simulink model "mCSControls_DG"  (R2012b)
settings: Solver=FixedStepDiscrete  StartTime=0.0  StopTime=10.0  RelTol=1e-3
values from neighbouring files (symbols this model uses):
  CDF2FThreshold = 45    [ControlCal_DG.m]
  CDF2TempThreshold = 20    [ControlCal_DG.m]
  delay = 5    [ControlCal_DG.m]
  DFThresh = 33    [ControlCal_DG.m]
  H = [90 90 90 90]    [ControlCal_DG.m]
  HeatTempThresh1 = 40    [ControlCal_DG.m]
  HeatTempThresh2 = 30    [ControlCal_DG.m]
  HeatTempThresh3 = 20    [ControlCal_DG.m]
  HStabilizationTime = 2*60    (= 120)    [ControlCal_DG.m]
  I_FAN = -1    [ControlCal_DG.m]
  I_VALVE = -1    [ControlCal_DG.m]
  initialSet = [1 1 1]    [ControlCal_DG.m]
  PBFTempThreshold = 30    [ControlCal_DG.m]
  PowerModeSwitchDelay = 30    [ControlCal_DG.m]
  SVocThresh = 550    [ControlCal_DG.m]
  T = [0 4 7 10]    [ControlCal_DG.m]
  Ts = 0.5    [ControlCal_DG.m]
  TSTempSetPoint = -2    [ControlCal_DG.m]
  TV1FThresh = 45    [ControlCal_DG.m]
  TV2FThresh = 60    [ControlCal_DG.m]
  VbatThresh = 22    [ControlCal_DG.m]
  VocDecRate = 0.5    [ControlCal_DG.m]
  VocIncrement = 5    [ControlCal_DG.m]
libraries: c2833xlib x29, simulink x23, c280xlib x11, idelinklib_tgtpref x1
(part 4 of 4)

== stateflow chart mCSControls_DG/Controls/Chart ==
  note: Variable 'count' is to find the time after the compressor has been switched off.
      | The heater is switched on if the time the compressor has been off > 45min.
      | Initally it's assigned a value > 45min to make sure heater runs at startup depending on ambient temp.
  state Running
    note: RelayOn is a global variable which controls when a relay can switch on.
        | This ensures only one relay switches on at a time and there is a 'delay' between multiple relays switching on.
    state StartupRelaysOff
      en,du:
      RelaysOP=RelaysOff;
      RelayOn=1;
      Pstatus=0;
    state PowerBatteryCheck
      en,du:
      [RelaysOP, Pstatus]=PowerModeSelection(RelaysOP,Inputs);
      count++;
    state PowerAvailable
      state PowerMonitor [parallel]
        settings: executionOrder=1
        state SolarPowerTesting
        state NormalOn
        note: Resetting TestVoc to threshold since it seems to run;
            | There is no guarantee TestVoc is the minimum Voc needed, it might be able to run at lower Voc too.
        state SwitchOff
          en,du: Pstatus=0;
        (default) -> NormalOn
        NormalOn -> SolarPowerTesting [order 2] : [RelaysOP.RS && Inputs.DriveParams.OP.OPFreq<DFThresh && RelaysOP.CRUN && CRUNOn]
        NormalOn -> NormalOn [order 1] : after(60,sec)[VocOffset>0]
            | {VocOffset=RelaysOP.RG*(VocOffset-VocDecRate)}
        SolarPowerTesting -> NormalOn [order 2] : after(20,sec){TestVoc = SVocThresh;}
        SolarPowerTesting -> SwitchOff [order 1] : after(20,sec)[powerSwitchCondition(RelaysOP, Inputs)]
        NormalOn -> SwitchOff [order 3] : [powerSwitchCondition(RelaysOP, Inputs)]
      state CompressorControl [parallel]
        settings: executionOrder=2
        state BeginCompressorOnSequence
        state switchOnHeater
          en:
          duration = heaterDuration(Inputs.Sensors.TA);
          du:
          RelaysOP.HEATER = 1;
        state SystemHeated
          en,du:
          RelaysOP.HEATER = 0;
          count = 0;
          CompOnCount = 0;
        state ValveCondenserCompressorControl
          state FanValveControl [parallel]
            settings: executionOrder=1
            note: FVOn ensures the Fault and Delay conditions in this substate are checked only when this valve switches on.
                | It is the local counterpart of the global variable RelayOn
            state FanValveOff
              en,du:
              RelaysOP.FV=0;
            state FanValveOn
              en:
              ILoadCurrent=Inputs.DCParams.Iload;
              RelaysOP.FV=1;
            state FanValveFault
              en:
              RelaysOP.FV=2;
            (default) -> Running.PowerAvailable.CompressorControl.ValveCondenserCompressorControl.FanValveControl.FanValveOff
            Running.PowerAvailable.CompressorControl.ValveCondenserCompressorControl.FanValveControl.FanValveOn -> Running.PowerAvailable.CompressorControl.ValveCondenserCompressorControl.FanValveControl.FanValveOff [order 1] : [~TempCondition(RelaysOP, Inputs)]{CompOnCount--; RelayOn=1;}
            Running.PowerAvailable.CompressorControl.ValveCondenserCompressorControl.FanValveControl.FanValveOff -> Running.PowerAvailable.CompressorControl.ValveCondenserCompressorControl.FanValveControl.FanValveOn : [RelayOn && TempCondition(RelaysOP, Inputs)]
                | {CompOnCount++; RelayOn=0;FVOn=0;}
            Running.PowerAvailable.CompressorControl.ValveCondenserCompressorControl.FanValveControl.FanValveOn -> Running.PowerAvailable.CompressorControl.ValveCondenserCompressorControl.FanValveControl.FanValveFault [order 3] : after(delay-1,sec)[~FVOn && Inputs.DCParams.Iload<ILoadCurrent+I_VALVE]{CompOnCount--; RelayOn=1;}
            Running.PowerAvailable.CompressorControl.ValveCondenserCompressorControl.FanValveControl.FanValveFault -> (junction 356) : after(105,sec){RelaysOP.FV=0}
            (junction 356) -> Running.PowerAvailable.CompressorControl.ValveCondenserCompressorControl.FanValveControl.FanValveOn : after(120,sec)[RelayOn]
                | {CompOnCount++; RelayOn=0; FVOn=0;}
            Running.PowerAvailable.CompressorControl.ValveCondenserCompressorControl.FanValveControl.FanValveOn -> Running.PowerAvailable.CompressorControl.ValveCondenserCompressorControl.FanValveControl.FanValveOn [order 2] : after(delay,sec)[~FVOn]{RelayOn=1; FVOn=1;}
          state ThermalStorageValve1Control [parallel]
            settings: executionOrder=2
            note: TV1On ensures the Fault and Delay conditions in this substate are checked only when this valve switches on.
                | It is the local counterpart of the global variable RelayOn
            state TV1ValveOff
              en,du:
              RelaysOP.TV1=0;
            state TESValveOn
              en,du:
              RelaysOP.TV1=1;
            (default) -> TV1ValveOff
            TESValveOn -> TV1ValveOff [order 1] : [~TV1TempOnCondition(RelaysOP, Inputs)]
                | {CompOnCount--; RelayOn=1;}
            TV1ValveOff -> TESValveOn : [RelayOn && TV1TempOnCondition(RelaysOP, Inputs)]
                | {CompOnCount++; RelayOn=0; TV1On=0;}
            TESValveOn -> TESValveOn [order 2] : after(delay,sec)[~TV1On]{RelayOn=1; TV1On=1;}
          state CompAndCondenserFan1Control [parallel]
            settings: executionOrder=3
            note: CDF1On and CRUNOn ensures the Fault and Delay conditions in this substate are checked only when this valve switches on.
                | It is the local counterpart of the global variable RelayOn
            state CompCondenserOff
              en,du:
              RelaysOP.CRUN=0;
              RelaysOP.RG2=0;
              RelaysOP.CDF1=0;
              count++;
            state CondenserFan1Fault
              en:
              RelaysOP.CDF1=2;
            state CondenserFan1On
              en:
              ILoadCurrent=Inputs.DCParams.Iload;
              RelaysOP.CDF1=1;
            state CompOn
              en: TestVoc = Inputs.DCParams.Voc
              du:
              RelaysOP.CRUN=1;
              count=0;
            (default) -> Running.PowerAvailable.CompressorControl.ValveCondenserCompressorControl.CompAndCondenserFan1Control.CompCondenserOff
            Running.PowerAvailable.CompressorControl.ValveCondenserCompressorControl.CompAndCondenserFan1Control.CompOn -> Running.PowerAvailable.CompressorControl.ValveCondenserCompressorControl.CompAndCondenserFan1Control.CompCondenserOff [order 2] : [CompOnCount==0]{RelayOn=1;}
            Running.PowerAvailable.CompressorControl.ValveCondenserCompressorControl.CompAndCondenserFan1Control.CompCondenserOff -> Running.PowerAvailable.CompressorControl.ValveCondenserCompressorControl.CompAndCondenserFan1Control.CondenserFan1On : [RelayOn && CompOnCount>0]
                | {RelayOn=0; CDF1On=0;}
            Running.PowerAvailable.CompressorControl.ValveCondenserCompressorControl.CompAndCondenserFan1Control.CondenserFan1On -> Running.PowerAvailable.CompressorControl.ValveCondenserCompressorControl.CompAndCondenserFan1Control.CondenserFan1Fault [order 3] : after(delay-1,sec)[~CDF1On && Inputs.DCParams.Iload<ILoadCurrent+I_FAN]{ RelayOn=1;}
            Running.PowerAvailable.CompressorControl.ValveCondenserCompressorControl.CompAndCondenserFan1Control.CondenserFan1On -> Running.PowerAvailable.CompressorControl.ValveCondenserCompressorControl.CompAndCondenserFan1Control.CondenserFan1On [order 1] : after(delay, sec)[~CDF1On]{RelayOn=1; CDF1On=1;}
            Running.PowerAvailable.CompressorControl.ValveCondenserCompressorControl.CompAndCondenserFan1Control.CondenserFan1Fault -> (junction 647) : after(105,sec){RelaysOP.CDF1=0;}
            (junction 647) -> Running.PowerAvailable.CompressorControl.ValveCondenserCompressorControl.CompAndCondenserFan1Control.CondenserFan1On : after(120,sec)[RelayOn]
                | {RelayOn=0; CDF1On=0;}
            Running.PowerAvailable.CompressorControl.ValveCondenserCompressorControl.CompAndCondenserFan1Control.CondenserFan1On -> Running.PowerAvailable.CompressorControl.ValveCondenserCompressorControl.CompAndCondenserFan1Control.CompOn [order 2] : [RelayOn]{RelayOn=0; CRUNOn=0;}
            Running.PowerAvailable.CompressorControl.ValveCondenserCompressorControl.CompAndCondenserFan1Control.CompOn -> Running.PowerAvailable.CompressorControl.ValveCondenserCompressorControl.CompAndCondenserFan1Control.CompOn [order 1] : after(1, sec)[~CRUNOn]
                | {RelayOn=1; CRUNOn=1; RelaysOP.RG2=RelaysOP.RG;}
          state CondenserFan2Control [parallel]
            settings: executionOrder=4
            note: CDF2On ensures the Fault and Delay conditions in this substate are checked only when this valve switches on.
                | It is the local counterpart of the global variable RelayOn
            state CondenserFan2Off
              en,du:
              RelaysOP.CDF2=0;
            state CondenserFan2Fault
              en:
              RelaysOP.CDF2=2;
            state CondenserFan2On
              en,du:
              ILoadCurrent=Inputs.DCParams.Iload;
              RelaysOP.CDF2=1;
            (default) -> Running.PowerAvailable.CompressorControl.ValveCondenserCompressorControl.CondenserFan2Control.CondenserFan2Off
            Running.PowerAvailable.CompressorControl.ValveCondenserCompressorControl.CondenserFan2Control.CondenserFan2On -> Running.PowerAvailable.CompressorControl.ValveCondenserCompressorControl.CondenserFan2Control.CondenserFan2Off [order 1] : [~CDF2Condition(RelaysOP, Inputs)]{RelayOn=1;}
            Running.PowerAvailable.CompressorControl.ValveCondenserCompressorControl.CondenserFan2Control.CondenserFan2Off -> Running.PowerAvailable.CompressorControl.ValveCondenserCompressorControl.CondenserFan2Control.CondenserFan2On : [RelayOn && CDF2Condition(RelaysOP, Inputs)]
                | {RelayOn=0; CDF2On=0;}
            Running.PowerAvailable.CompressorControl.ValveCondenserCompressorControl.CondenserFan2Control.CondenserFan2On -> Running.PowerAvailable.CompressorControl.ValveCondenserCompressorControl.CondenserFan2Control.CondenserFan2Fault [order 3] : after(delay-1,sec)[~CDF2On && Inputs.DCParams.Iload<ILoadCurrent+I_FAN]{ RelayOn=1;}
            Running.PowerAvailable.CompressorControl.ValveCondenserCompressorControl.CondenserFan2Control.CondenserFan2Fault -> (junction 433) : after(105,sec){RelaysOP.CDF2=0;}
            (junction 433) -> Running.PowerAvailable.CompressorControl.ValveCondenserCompressorControl.CondenserFan2Control.CondenserFan2On : after(120,sec)[RelayOn]
                | {RelayOn=0; CDF2On=0;}
            Running.PowerAvailable.CompressorControl.ValveCondenserCompressorControl.CondenserFan2Control.CondenserFan2On -> Running.PowerAvailable.CompressorControl.ValveCondenserCompressorControl.CondenserFan2Control.CondenserFan2On [order 2] : after(delay,sec)[~CDF2On]{RelayOn=1; CDF2On=1;}
          note: CompOnCount keeps count of how many relays are On.
              | If it is greater than 1, the compressor switches on.
        (default) -> Running.PowerAvailable.CompressorControl.BeginCompressorOnSequence
        Running.PowerAvailable.CompressorControl.ValveCondenserCompressorControl -> Running.PowerAvailable.CompressorControl.BeginCompressorOnSequence : [count>2700/Ts]
        Running.PowerAvailable.CompressorControl.BeginCompressorOnSequence -> Running.PowerAvailable.CompressorControl.SystemHeated [order 2] : after(delay,sec)
        Running.PowerAvailable.CompressorControl.BeginCompressorOnSequence -> Running.PowerAvailable.CompressorControl.switchOnHeater [order 1] : [Inputs.Sensors.TA<HeatTempThresh1 && count>2700/Ts]
        Running.PowerAvailable.CompressorControl.switchOnHeater -> Running.PowerAvailable.CompressorControl.SystemHeated : after(duration, sec)
        Running.PowerAvailable.CompressorControl.SystemHeated -> Running.PowerAvailable.CompressorControl.ValveCondenserCompressorControl : after(delay, sec)
      state HumidityControl [parallel]
        settings: executionOrder=3
        state HumidityPumpOff
          en,du:
          RelaysOP.PUMP=0;
          RelaysOP.PV=0;
        note: HOn ensures the Fault and Delay conditions in this substate are checked only when this valve switches on.
            | It is the local counterpart of the global variable RelayOn
        state HumidityPumpOn
          en,du:
          RelaysOP.PV=1;
          RelaysOP.PUMP=1;
        (default) -> Running.PowerAvailable.HumidityControl.HumidityPumpOff
        Running.PowerAvailable.HumidityControl.HumidityPumpOn -> Running.PowerAvailable.HumidityControl.HumidityPumpOff [order 2] : [~HCondition(Inputs)]{RelayOn=1;}
        Running.PowerAvailable.HumidityControl.HumidityPumpOff -> Running.PowerAvailable.HumidityControl.HumidityPumpOn : [RelayOn && HCondition(Inputs)]
            | {RelayOn=0; HOn=0;}
        Running.PowerAvailable.HumidityControl.HumidityPumpOn -> Running.PowerAvailable.HumidityControl.HumidityPumpOn [order 1] : after(delay,sec)[~HOn]{RelayOn=1; HOn=1;}
      state FanControl [parallel]
        settings: executionOrder=4
        state FanOff
          en,du:
          RelaysOP.F1=0
          RelaysOP.F2=0;
        note: FOn ensures the Fault and Delay conditions in this substate are checked only when this valve switches on.
            | It is the local counterpart of the global variable RelayOn
        state FanFault
          en:
          RelaysOP.F1=2;
          RelaysOP.F2=2;
        state Fan2Off
          en,du:
          ILoadCurrent=Inputs.DCParams.Iload;
          RelaysOP.F1=1;
          RelaysOP.F2=0;
        state FansOn
          en,du:
          RelaysOP.F1=1;
          RelaysOP.F2=1;
        (default) -> Running.PowerAvailable.FanControl.FanOff
        Running.PowerAvailable.FanControl.Fan2Off -> Running.PowerAvailable.FanControl.FanOff [order 1] : [~RelaysOP.FV]{RelayOn=1;}
        Running.PowerAvailable.FanControl.FanOff -> Running.PowerAvailable.FanControl.Fan2Off : [RelayOn && RelaysOP.FV==1]
            | {RelayOn=0; FOn=0;}
        Running.PowerAvailable.FanControl.Fan2Off -> Running.PowerAvailable.FanControl.FanFault [order 3] : after(delay-1,sec)[~FOn && Inputs.DCParams.Iload<ILoadCurrent+I_FAN]{ RelayOn=1;}
        Running.PowerAvailable.FanControl.Fan2Off -> Running.PowerAvailable.FanControl.FansOn [order 4] : after(3*60,sec)[RelaysOP.FV==1]
        Running.PowerAvailable.FanControl.FanFault -> (junction 439) : after(105,sec){RelaysOP.F1=0; RelaysOP.F2=0;}
        (junction 439) -> Running.PowerAvailable.FanControl.Fan2Off : after(120,sec)[RelayOn]
            | {RelayOn=0; FOn=0;}
        Running.PowerAvailable.FanControl.FansOn -> Running.PowerAvailable.FanControl.Fan2Off : after(1*60,sec)
        Running.PowerAvailable.FanControl.Fan2Off -> Running.PowerAvailable.FanControl.Fan2Off [order 2] : after(delay,sec)[~FOn]{RelayOn=1; FOn=1;}
      state PanelBoxFanControl [parallel]
        settings: executionOrder=5
        state PanelBoxFanOff
          en,du:
          RelaysOP.PBF=0
        note: PBFOn ensures the Fault and Delay conditions in this substate are checked only when this valve switches on.
            | It is the local counterpart of the global variable RelayOn
        note: 0.5 is for Hysteresis in temperature control
        state PanelBoxFanOn
          en,du:
          RelaysOP.PBF=1;
        (default) -> Running.PowerAvailable.PanelBoxFanControl.PanelBoxFanOff
        Running.PowerAvailable.PanelBoxFanControl.PanelBoxFanOn -> Running.PowerAvailable.PanelBoxFanControl.PanelBoxFanOff [order 1] : [Inputs.Sensors.TA<PBFTempThreshold-0.5]{RelayOn=1;}
        Running.PowerAvailable.PanelBoxFanControl.PanelBoxFanOff -> Running.PowerAvailable.PanelBoxFanControl.PanelBoxFanOn : [RelayOn && Inputs.Sensors.TA>PBFTempThreshold]
            | {RelayOn=0; PBFOn=0;}
        Running.PowerAvailable.PanelBoxFanControl.PanelBoxFanOn -> Running.PowerAvailable.PanelBoxFanControl.PanelBoxFanOn [order 2] : after(delay,sec)[~PBFOn]{RelayOn=1; PBFOn=1;}
    state RelaysOff
      en,du:
      RelaysOP=RelaysOff;
      RelayOn=1;
    state BatteryAvailable
      state PowerMonitor [parallel]
        settings: executionOrder=1
        state PowerNotAvailable
          en,du: count++
        state PowerAvailable
          en,du: Pstatus=1;
        (default) -> Running.BatteryAvailable.PowerMonitor.PowerNotAvailable
        Running.BatteryAvailable.PowerMonitor.PowerNotAvailable -> Running.BatteryAvailable.PowerMonitor.PowerNotAvailable [order 2] : after(60,sec)[VocOffset>0]
            | {VocOffset=VocOffset-VocDecRate}
        Running.BatteryAvailable.PowerMonitor.PowerNotAvailable -> Running.BatteryAvailable.PowerMonitor.PowerAvailable [order 1] : [powerOnCondition(RelaysOP, Inputs)]
      state HumidityControl [parallel]
        settings: executionOrder=2
        state HumidityPumpOff
          en,du:
          RelaysOP.PUMP=0;
          RelaysOP.PV=0;
        note: HOn ensures the Fault and Delay conditions in this substate are checked only when this valve switches on.
            | It is the local counterpart of the global variable RelayOn
        state HumidityPumpOn
          en,du:
          RelaysOP.PV=1;
          RelaysOP.PUMP=1;
        (default) -> Running.BatteryAvailable.HumidityControl.HumidityPumpOff
        Running.BatteryAvailable.HumidityControl.HumidityPumpOn -> Running.BatteryAvailable.HumidityControl.HumidityPumpOff [order 2] : [~HCondition(Inputs)]{RelayOn=1;}
        Running.BatteryAvailable.HumidityControl.HumidityPumpOff -> Running.BatteryAvailable.HumidityControl.HumidityPumpOn : [RelayOn && HCondition(Inputs)]
            | {RelayOn=0; HOn=0;}
        Running.BatteryAvailable.HumidityControl.HumidityPumpOn -> Running.BatteryAvailable.HumidityControl.HumidityPumpOn [order 1] : after(delay,sec)[~HOn]{RelayOn=1; HOn=1;}
      state FanControl [parallel]
        settings: executionOrder=3
        (history)
        note: FOn ensures the Fault and Delay conditions in this substate are checked only when this valve switches on.
            | It is the local counterpart of the global variable RelayOn
        state FanOff
          en,du:
          RelaysOP.F1=0
          RelaysOP.F2=0;
        state FanConditionalOff
          en,du:
          RelaysOP.F1=0;
          RelaysOP.F2=0;
        state FanConditionalOn
          en:CurrentH1Temp=Inputs.Sensors.TH1;
          du:
          RelaysOP.F1=1;
          RelaysOP.F2=0;
        note: In Battery Mode, if Temperature of the Holding is greater than setpoint,
            | switch on the fan, wait for 5 min to see if temp reduces, but if not,
            | switch off the fan.
        (default) -> Running.BatteryAvailable.FanControl.FanOff
        Running.BatteryAvailable.FanControl.FanOff -> FanConditionalOn : [RelayOn && TempCheck(RelaysOP, Inputs)]
            | {RelayOn=0; FOn=0;}
        FanConditionalOff -> Running.BatteryAvailable.FanControl.FanOff [order 1] : [~TempCheck(RelaysOP, Inputs)]{RelayOn=1;}
        FanConditionalOn -> Running.BatteryAvailable.FanControl.FanOff [order 1] : [~TempCheck(RelaysOP, Inputs)]{RelayOn=1;}
        FanConditionalOn -> FanConditionalOff [order 3] : after(5*60,sec)
            | [Inputs.Sensors.TH1>CurrentH1Temp]
        FanConditionalOff -> FanConditionalOn [order 2] : after(4*60,sec)
        FanConditionalOn -> FanConditionalOn [order 2] : after(delay,sec)[~FOn]{RelayOn=1; FOn=1;}
      state PanelBoxFanControl [parallel]
        settings: executionOrder=4
        state PanelBoxFanOff
          en,du:
          RelaysOP.PBF=0
        note: PBFOn ensures the Fault and Delay conditions in this substate are checked only when this valve switches on.
            | It is the local counterpart of the global variable RelayOn
        note: 0.5 is for Hysteresis in temperature control
        state PanelBoxFanOn
          en,du:
          RelaysOP.PBF=1;
        (default) -> Running.BatteryAvailable.PanelBoxFanControl.PanelBoxFanOff
        Running.BatteryAvailable.PanelBoxFanControl.PanelBoxFanOn -> Running.BatteryAvailable.PanelBoxFanControl.PanelBoxFanOff [order 1] : [Inputs.Sensors.TA<PBFTempThreshold-0.5]{RelayOn=1;}
        Running.BatteryAvailable.PanelBoxFanControl.PanelBoxFanOff -> Running.BatteryAvailable.PanelBoxFanControl.PanelBoxFanOn : [RelayOn && Inputs.Sensors.TA>PBFTempThreshold]
            | {RelayOn=0; PBFOn=0;}
        Running.BatteryAvailable.PanelBoxFanControl.PanelBoxFanOn -> Running.BatteryAvailable.PanelBoxFanControl.PanelBoxFanOn [order 2] : after(delay,sec)[~PBFOn]{RelayOn=1; PBFOn=1;}
    state DieselMode
      state PowerMonitor [parallel]
        settings: executionOrder=1
        state TestingDG
        state PowerNotAvailable
        state SwitchOffDiesel
          en,du: RelaysOP.DGOFF=1;
        state PowerAvailable
          en,du:
          RelaysOP.DGOFF=0;
          Pstatus=1;
        (default) -> Running.DieselMode.PowerMonitor.PowerNotAvailable
        Running.DieselMode.PowerMonitor.PowerNotAvailable -> TestingDG [order 3] : [RelaysOP.CRUN==1 && Inputs.DriveParams.OP.OPFreq<DFThresh]
        Running.DieselMode.PowerMonitor.PowerNotAvailable -> Running.DieselMode.PowerMonitor.PowerNotAvailable [order 2] : after(60,sec)[VocOffset>0]
            | {VocOffset=VocOffset-VocDecRate}
        TestingDG -> Running.DieselMode.PowerMonitor.PowerNotAvailable [order 1] : after(20,sec)[Inputs.DriveParams.OP.OPFreq>DFThresh]
        TestingDG -> SwitchOffDiesel [order 2] : after(20,sec)
        Running.DieselMode.PowerMonitor.PowerNotAvailable -> SwitchOffDiesel [order 1] : [powerOnCondition(RelaysOP, Inputs) || Inputs.DCParams.Vbat<VbatThresh]
        SwitchOffDiesel -> Running.DieselMode.PowerMonitor.PowerAvailable : after(4,sec)
      state CompressorControl [parallel]
        settings: executionOrder=2
        state BeginCompressorOnSequence
        state switchOnHeater
          en:
          duration = heaterDuration(Inputs.Sensors.TA);
          du:
          RelaysOP.HEATER = 1;
        state SystemHeated
          en,du:
          RelaysOP.HEATER = 0;
          count = 0;
          CompOnCount = 0;
        state ValveCondenserCompressorControl
          state FanValveControl [parallel]
            settings: executionOrder=1
            note: FVOn ensures the Fault and Delay conditions in this substate are checked only when this valve switches on.
                | It is the local counterpart of the global variable RelayOn
            state FanValveOff
              en,du:
              RelaysOP.FV=0;
            state FanValveOn
              en:
              ILoadCurrent=Inputs.DCParams.Iload;
              RelaysOP.FV=1;
            state FanValveFault
              en:
              RelaysOP.FV=2;
            (default) -> Running.DieselMode.CompressorControl.ValveCondenserCompressorControl.FanValveControl.FanValveOff
            Running.DieselMode.CompressorControl.ValveCondenserCompressorControl.FanValveControl.FanValveOn -> Running.DieselMode.CompressorControl.ValveCondenserCompressorControl.FanValveControl.FanValveOff [order 1] : [~TempCondition(RelaysOP, Inputs)]{CompOnCount--; RelayOn=1;}
            Running.DieselMode.CompressorControl.ValveCondenserCompressorControl.FanValveControl.FanValveOff -> Running.DieselMode.CompressorControl.ValveCondenserCompressorControl.FanValveControl.FanValveOn : [RelayOn && TempCondition(RelaysOP, Inputs)]
                | {CompOnCount++; RelayOn=0;FVOn=0;}
            Running.DieselMode.CompressorControl.ValveCondenserCompressorControl.FanValveControl.FanValveOn -> Running.DieselMode.CompressorControl.ValveCondenserCompressorControl.FanValveControl.FanValveFault [order 3] : after(delay-1,sec)[~FVOn && Inputs.DCParams.Iload<ILoadCurrent+I_VALVE]{CompOnCount--; RelayOn=1;}
            Running.DieselMode.CompressorControl.ValveCondenserCompressorControl.FanValveControl.FanValveFault -> (junction 796) : after(105,sec){RelaysOP.FV=0}
            (junction 796) -> Running.DieselMode.CompressorControl.ValveCondenserCompressorControl.FanValveControl.FanValveOn : after(120,sec)[RelayOn]
                | {CompOnCount++; RelayOn=0; FVOn=0;}
            Running.DieselMode.CompressorControl.ValveCondenserCompressorControl.FanValveControl.FanValveOn -> Running.DieselMode.CompressorControl.ValveCondenserCompressorControl.FanValveControl.FanValveOn [order 2] : after(delay,sec)[~FVOn]{RelayOn=1; FVOn=1;}
          state CompAndCondenserFan1Control [parallel]
            settings: executionOrder=2
            state CompCondenserOff
              en,du:
              RelaysOP.DGOFF=0;
              RelaysOP.RDG1=0;
              RelaysOP.CRUN=0;
              RelaysOP.RG2=0;
              RelaysOP.CDF1=0;
              count++;
            note: CDF1On and CRUNOn ensures the Fault and Delay conditions in this substate are checked only when this valve switches on.
                | It is the local counterpart of the global variable RelayOn
            state CondenserFan1Fault
              en:
              RelaysOP.CDF1=2;
            state CondenserFan1On
              en:
              ILoadCurrent=Inputs.DCParams.Iload;
              RelaysOP.CDF1=1;
            state DieselOff
              en,du:
              RelaysOP.DGOFF=1;
            state DieselOn
              en,du:
              RelaysOP.DGON=1;
              RelaysOP.RDG1=1;
            state CompOn
              en,du:
              RelaysOP.DGON=0;
              RelaysOP.CRUN=1;
              count=0;
            (default) -> Running.DieselMode.CompressorControl.ValveCondenserCompressorControl.CompAndCondenserFan1Control.CompCondenserOff
            Running.DieselMode.CompressorControl.ValveCondenserCompressorControl.CompAndCondenserFan1Control.DieselOff -> Running.DieselMode.CompressorControl.ValveCondenserCompressorControl.CompAndCondenserFan1Control.CompCondenserOff : after(4,sec)
            Running.DieselMode.CompressorControl.ValveCondenserCompressorControl.CompAndCondenserFan1Control.CompCondenserOff -> Running.DieselMode.CompressorControl.ValveCondenserCompressorControl.CompAndCondenserFan1Control.CondenserFan1On : [RelayOn && CompOnCount>0]
                | {RelayOn=0; CDF1On=0;}
            Running.DieselMode.CompressorControl.ValveCondenserCompressorControl.CompAndCondenserFan1Control.CondenserFan1On -> Running.DieselMode.CompressorControl.ValveCondenserCompressorControl.CompAndCondenserFan1Control.CondenserFan1Fault [order 3] : after(delay-1,sec)[~CDF1On && Inputs.DCParams.Iload<ILoadCurrent+I_FAN]{ RelayOn=1;}
            Running.DieselMode.CompressorControl.ValveCondenserCompressorControl.CompAndCondenserFan1Control.CondenserFan1On -> Running.DieselMode.CompressorControl.ValveCondenserCompressorControl.CompAndCondenserFan1Control.CondenserFan1On [order 1] : after(delay, sec)[~CDF1On]{RelayOn=1; CDF1On=1;}
            Running.DieselMode.CompressorControl.ValveCondenserCompressorControl.CompAndCondenserFan1Control.CondenserFan1Fault -> (junction 825) : after(105,sec){RelaysOP.CDF1=0;}
            (junction 825) -> Running.DieselMode.CompressorControl.ValveCondenserCompressorControl.CompAndCondenserFan1Control.CondenserFan1On : after(120,sec)[RelayOn]
                | {RelayOn=0; CDF1On=0;}
            Running.DieselMode.CompressorControl.ValveCondenserCompressorControl.CompAndCondenserFan1Control.CondenserFan1On -> Running.DieselMode.CompressorControl.ValveCondenserCompressorControl.CompAndCondenserFan1Control.DieselOn [order 2] : [RelayOn]{RelayOn=0; CRUNOn=0;}
            Running.DieselMode.CompressorControl.ValveCondenserCompressorControl.CompAndCondenserFan1Control.CompOn -> Running.DieselMode.CompressorControl.ValveCondenserCompressorControl.CompAndCondenserFan1Control.DieselOff [order 2] : [CompOnCount==0]{RelayOn=1;}
            Running.DieselMode.CompressorControl.ValveCondenserCompressorControl.CompAndCondenserFan1Control.DieselOn -> Running.DieselMode.CompressorControl.ValveCondenserCompressorControl.CompAndCondenserFan1Control.CompOn : after(4,sec)
            Running.DieselMode.CompressorControl.ValveCondenserCompressorControl.CompAndCondenserFan1Control.CompOn -> Running.DieselMode.CompressorControl.ValveCondenserCompressorControl.CompAndCondenserFan1Control.CompOn [order 1] : after(1, sec)[~CRUNOn]
                | {RelayOn=1; CRUNOn=1; RelaysOP.RG2=1;}
          state CondenserFan2Control [parallel]
            settings: executionOrder=3
            note: CDF2On ensures the Fault and Delay conditions in this substate are checked only when this valve switches on.
                | It is the local counterpart of the global variable RelayOn
            state CondenserFan2Off
              en,du:
              RelaysOP.CDF2=0;
            state CondenserFan2Fault
              en:
              RelaysOP.CDF2=2;
            state CondenserFan2On
              en,du:
              ILoadCurrent=Inputs.DCParams.Iload;
              RelaysOP.CDF2=1;
            (default) -> Running.DieselMode.CompressorControl.ValveCondenserCompressorControl.CondenserFan2Control.CondenserFan2Off
            Running.DieselMode.CompressorControl.ValveCondenserCompressorControl.CondenserFan2Control.CondenserFan2On -> Running.DieselMode.CompressorControl.ValveCondenserCompressorControl.CondenserFan2Control.CondenserFan2Off [order 1] : [~CDF2Condition(RelaysOP, Inputs)]{RelayOn=1;}
            Running.DieselMode.CompressorControl.ValveCondenserCompressorControl.CondenserFan2Control.CondenserFan2Off -> Running.DieselMode.CompressorControl.ValveCondenserCompressorControl.CondenserFan2Control.CondenserFan2On : [RelayOn && CDF2Condition(RelaysOP, Inputs)]
                | {RelayOn=0; CDF2On=0;}
            Running.DieselMode.CompressorControl.ValveCondenserCompressorControl.CondenserFan2Control.CondenserFan2On -> Running.DieselMode.CompressorControl.ValveCondenserCompressorControl.CondenserFan2Control.CondenserFan2Fault [order 3] : after(delay-1,sec)[~CDF2On && Inputs.DCParams.Iload<ILoadCurrent+I_FAN]{ RelayOn=1;}
            Running.DieselMode.CompressorControl.ValveCondenserCompressorControl.CondenserFan2Control.CondenserFan2Fault -> (junction 841) : after(105,sec){RelaysOP.CDF2=0;}
            (junction 841) -> Running.DieselMode.CompressorControl.ValveCondenserCompressorControl.CondenserFan2Control.CondenserFan2On : after(120,sec)[RelayOn]
                | {RelayOn=0; CDF2On=0;}
            Running.DieselMode.CompressorControl.ValveCondenserCompressorControl.CondenserFan2Control.CondenserFan2On -> Running.DieselMode.CompressorControl.ValveCondenserCompressorControl.CondenserFan2Control.CondenserFan2On [order 2] : after(delay,sec)[~CDF2On]{RelayOn=1; CDF2On=1;}
          note: CompOnCount keeps count of how many relays are On.
              | If it is greater than 1, the compressor switches on.
        (default) -> Running.DieselMode.CompressorControl.BeginCompressorOnSequence
        Running.DieselMode.CompressorControl.ValveCondenserCompressorControl -> Running.DieselMode.CompressorControl.BeginCompressorOnSequence : [count>2700/Ts]
        Running.DieselMode.CompressorControl.BeginCompressorOnSequence -> Running.DieselMode.CompressorControl.SystemHeated [order 2] : after(delay,sec)
        Running.DieselMode.CompressorControl.BeginCompressorOnSequence -> Running.DieselMode.CompressorControl.switchOnHeater [order 1] : [Inputs.Sensors.TA<HeatTempThresh1 && count>2700/Ts]
        Running.DieselMode.CompressorControl.switchOnHeater -> Running.DieselMode.CompressorControl.SystemHeated : after(duration, sec)
        Running.DieselMode.CompressorControl.SystemHeated -> Running.DieselMode.CompressorControl.ValveCondenserCompressorControl : after(delay, sec)
      state HumidityControl [parallel]
        settings: executionOrder=3
        state HumidityPumpOff
          en,du:
          RelaysOP.PUMP=0;
          RelaysOP.PV=0;
        note: HOn ensures the Fault and Delay conditions in this substate are checked only when this valve switches on.
            | It is the local counterpart of the global variable RelayOn
        state HumidityPumpOn
          en,du:
          RelaysOP.PV=1;
          RelaysOP.PUMP=1;
        (default) -> Running.DieselMode.HumidityControl.HumidityPumpOff
        Running.DieselMode.HumidityControl.HumidityPumpOn -> Running.DieselMode.HumidityControl.HumidityPumpOff [order 2] : [~HCondition(Inputs)]{RelayOn=1;}
        Running.DieselMode.HumidityControl.HumidityPumpOff -> Running.DieselMode.HumidityControl.HumidityPumpOn : [RelayOn && HCondition(Inputs)]
            | {RelayOn=0; HOn=0;}
        Running.DieselMode.HumidityControl.HumidityPumpOn -> Running.DieselMode.HumidityControl.HumidityPumpOn [order 1] : after(delay,sec)[~HOn]{RelayOn=1; HOn=1;}
      state FanControl [parallel]
        settings: executionOrder=4
        state FanOff
          en,du:
          RelaysOP.F1=0
          RelaysOP.F2=0;
        note: FOn ensures the Fault and Delay conditions in this substate are checked only when this valve switches on.
            | It is the local counterpart of the global variable RelayOn
        state FanFault
          en:
          RelaysOP.F1=2;
          RelaysOP.F2=2;
        state Fan2Off
          en,du:
          ILoadCurrent=Inputs.DCParams.Iload;
          RelaysOP.F1=1;
          RelaysOP.F2=0;
        state FansOn
          en,du:
          RelaysOP.F1=1;
          RelaysOP.F2=1;
        (default) -> Running.DieselMode.FanControl.FanOff
        Running.DieselMode.FanControl.Fan2Off -> Running.DieselMode.FanControl.FanOff [order 1] : [~RelaysOP.FV]{RelayOn=1;}
        Running.DieselMode.FanControl.FanOff -> Running.DieselMode.FanControl.Fan2Off : [RelayOn && RelaysOP.FV==1]
            | {RelayOn=0; FOn=0;}
        Running.DieselMode.FanControl.Fan2Off -> Running.DieselMode.FanControl.FanFault [order 3] : after(delay-1,sec)[~FOn && Inputs.DCParams.Iload<ILoadCurrent+I_FAN]{ RelayOn=1;}
        Running.DieselMode.FanControl.Fan2Off -> Running.DieselMode.FanControl.FansOn [order 4] : after(3*60,sec)[RelaysOP.FV==1]
        Running.DieselMode.FanControl.FanFault -> (junction 926) : after(105,sec){RelaysOP.F1=0; RelaysOP.F2=0;}
        (junction 926) -> Running.DieselMode.FanControl.Fan2Off : after(120,sec)[RelayOn]
            | {RelayOn=0; FOn=0;}
        Running.DieselMode.FanControl.FansOn -> Running.DieselMode.FanControl.Fan2Off : after(1*60,sec)
        Running.DieselMode.FanControl.Fan2Off -> Running.DieselMode.FanControl.Fan2Off [order 2] : after(delay,sec)[~FOn]{RelayOn=1; FOn=1;}
      state PanelBoxFanControl [parallel]
        settings: executionOrder=5
        state PanelBoxFanOff
          en,du:
          RelaysOP.PBF=0
        note: PBFOn ensures the Fault and Delay conditions in this substate are checked only when this valve switches on.
            | It is the local counterpart of the global variable RelayOn
        note: PBF always on in DG mode to cool rectifier
        state PanelBoxFanOn
          en,du:
          RelaysOP.PBF=1;
        (default) -> Running.DieselMode.PanelBoxFanControl.PanelBoxFanOff
        Running.DieselMode.PanelBoxFanControl.PanelBoxFanOff -> Running.DieselMode.PanelBoxFanControl.PanelBoxFanOn : [RelayOn]
            | {RelayOn=0; PBFOn=0;}
        Running.DieselMode.PanelBoxFanControl.PanelBoxFanOn -> Running.DieselMode.PanelBoxFanControl.PanelBoxFanOn : after(delay,sec)[~PBFOn]{RelayOn=1; PBFOn=1;}
      state BatteryChargeControl [parallel]
        settings: executionOrder=6
        state BatteryChargerOff
          en,du:
          RelaysOP.DGBATCHG=0
        state DieselOn
          en,du:
          RelaysOP.DGBATCHG=0;
        state BatteryChargerOn
          en,du:
          RelaysOP.DGBATCHG=1;
        (default) -> Running.DieselMode.BatteryChargeControl.BatteryChargerOff
        Running.DieselMode.BatteryChargeControl.BatteryChargerOn -> Running.DieselMode.BatteryChargeControl.BatteryChargerOff : [Inputs.DriveParams.OP.OPFreq<DFThresh]
        Running.DieselMode.BatteryChargeControl.DieselOn -> Running.DieselMode.BatteryChargeControl.BatteryChargerOff [order 2] : [Inputs.DriveParams.OP.OPFreq<DFThresh]
        Running.DieselMode.BatteryChargeControl.BatteryChargerOff -> Running.DieselMode.BatteryChargeControl.DieselOn : [Inputs.DriveParams.OP.OPFreq>DFThresh]
        Running.DieselMode.BatteryChargeControl.DieselOn -> Running.DieselMode.BatteryChargeControl.BatteryChargerOn [order 1] : after(30,sec)
    state DGBatteryChargeControl
      state DieselOn
        en,du:
        RelaysOP.DGON=1
        RelaysOP.DGBATCHG=0
      state BatteryChargerOn
        en,du:
        RelaysOP.DGON=0;
        RelaysOP.DGBATCHG=1;
        RelaysOP.PBF=1;
      state DieselOff
        en,du:
        RelaysOP.DGOFF=0;
        RelaysOP.PBF=0;
      state BatteryChargerOff
        en,du:
        RelaysOP.DGBATCHG=0;
        RelaysOP.DGOFF=1;
      (default) -> Running.DGBatteryChargeControl.DieselOn
      Running.DGBatteryChargeControl.DieselOn -> Running.DGBatteryChargeControl.BatteryChargerOn : after(4,sec)
      Running.DGBatteryChargeControl.BatteryChargerOn -> Running.DGBatteryChargeControl.BatteryChargerOff : after(15*60,sec)
      Running.DGBatteryChargeControl.BatteryChargerOff -> Running.DGBatteryChargeControl.DieselOff : after(4,sec)
    (default) -> StartupRelaysOff
    StartupRelaysOff -> PowerBatteryCheck : after(delay+15,sec)
    PowerBatteryCheck -> Running.PowerAvailable [order 1] : [Pstatus && Inputs.DCParams.Vbat>VbatThresh]
    PowerBatteryCheck -> DGBatteryChargeControl [order 3] : [Inputs.DCParams.Vbat<VbatThresh]
    Running.PowerAvailable -> RelaysOff : [~Pstatus || Inputs.DCParams.Vbat<VbatThresh]
    RelaysOff -> PowerBatteryCheck : after(PowerModeSwitchDelay,sec)
    DGBatteryChargeControl -> PowerBatteryCheck : after(16*60,sec)
    PowerBatteryCheck -> BatteryAvailable [order 2] : [~Pstatus && Inputs.DCParams.Vbat>VbatThresh]
    BatteryAvailable -> RelaysOff [order 1] : [Pstatus || Inputs.DCParams.Vbat<VbatThresh]
    DieselMode -> RelaysOff : [Pstatus]
    BatteryAvailable -> DieselMode [order 2] : after(5*60,sec)[Diesel(RelaysOP,Inputs)]
  state Off
    en,du:
    RelaysOP=RelaysOff;
    count++;
  note: Switching off DG set if its on
  state DGOff
    en,du:
    RelaysOP.DGOFF=1;
  (default) -> Off : {count=3000/Ts;}
  Off -> Running : [Inputs.EEPROM.P1 && Inputs.PowerIP.PowerIP]
  Running -> DGOff : [~Inputs.EEPROM.P1 || ~Inputs.PowerIP.PowerIP]
  DGOff -> Off : after(4,sec)
  data: R1 function_output Bus: Relays; R function_input Bus: Relays; In function_input Bus: Inputs; PS function_output double size=1; R function_input Bus: Relays; In function_input Bus: Inputs; y function_output double; TA function_input double; dur function_output double; R function_input Bus: Relays; y function_output double; In function_input Bus: Inputs; R function_input Bus: Relays; In function_input Bus: Inputs; y function_output double size=1 =0; R function_input Bus: Relays; In function_input Bus: Inputs; y function_output double; In function_input Bus: Inputs; y function_output double; R function_input Bus: Relays; In function_input Bus: Inputs; y function_output double; In function_input Bus: Inputs; y function_output double; R function_input Bus: Relays; In function_input Bus: Inputs; y function_output double; R function_input Bus: Relays; In function_input Bus: Inputs; y function_output double; TA function_input double; dur function_output double; R function_input Bus: Relays; y function_output double; In function_input Bus: Inputs; R function_input Bus: Relays; In function_input Bus: Inputs; y function_output double; In function_input Bus: Inputs; y function_output double; R function_input Bus: Relays; In function_input Bus: Inputs; y function_output double; Inputs input Bus: Inputs; RelaysOff input Bus: Relays; RelaysOP output Bus: Relays; Pstatus local double size=1 =0; HeatTempThresh1 parameter double; PowerModeSwitchDelay parameter double; VbatThresh parameter double; delay parameter double; duration local double; SVocThresh parameter double size=1; DFThresh parameter double size=1; HeatTempThresh2 parameter double size=1; count local double size=1 =0; Ts parameter double size=1; CompOnCount local double size=1 =0; RelayOn local double size=1 =1; TV1FThresh parameter double; TSTempSetPoint parameter double; TV2FThresh parameter double; T parameter double; CDF2TempThreshold parameter double; H parameter double; HStabilizationTime parameter double; PBFTempThreshold parameter double; CurrentH1Temp local double; CDF2FThreshold parameter double; HeatTempThresh3 parameter double size=1; ILoadCurrent local double; I_VALVE parameter double; FVOn local double; TV1On local double; TV2On local double; CDF1On local double; CRUNOn local double; CDF2On local double; HOn local double; FOn local double; PBFOn local double; I_FAN parameter double; DamperCount local double =0; DamperOn local double; VocIncrement parameter double; VocDecRate parameter double; VocOffset local double =0; TestVoc local double
  function [R1,PS]=PowerModeSelection(R,In):
    | function [R1,PS]=PowerModeSelection(R,In)
    | 
    | % Output Initialization
    | R1=R;
    | PS=0;
    | 
    | %Required Variables
    | mode = In.EEPROM.M1;
    | SolarVoc = In.DCParams.Voc;
    | gridAvail = In.DCParams.GRID;
    | driveFreq = In.DriveParams.OP.OPFreq;
    | 
    | %Info
    | % mode==1=>Auto
    | % mode==2=>Solar
    | % mode==3=>Grid
    | 
    | if (((mode==2)||(mode==1)) && (SolarVoc>SVocThresh+VocOffset))
    |     R1.RS=1;
    |     PS=1;
    | else
    |     R1.RS=0;
    | end
    | 
    | if (gridAvail && ~R1.RS && (mode~=2))
    |     R1.RG=1;
    |     PS=1;
    | else
    |     R1.RG=0;
    | end
  function y=powerSwitchCondition(R, In):
    | function y=powerSwitchCondition(R, In)
    |  
    | y=0;
    | 
    | if (R.RS)
    |     % operating in Solar
    |     
    |     if (In.EEPROM.M1==3)
    |         % switched mode to Grid
    |         y=1;
    |     end 
    |     
    |     if (In.DriveParams.OP.OPFreq<DFThresh && R.CRUN && CRUNOn)
    |         % not enough power output in Solar
    |         % (CRUNOn will make sure we wait for some sec after commanding CRUN to check this condition)
    |         y=1;
    |         VocOffset = max(VocOffset,(TestVoc-SVocThresh)) + VocIncrement;
    |     end
    | end
    | 
    | 
    | if (R.RG)
    |     % operating in Grid
    |     
    |     if (In.EEPROM.M1==2)
    |         % switched mode to Solar
    |         VocOffset = 0;
    |         y=1;
    |     end
    |     
    |     if (~In.DCParams.GRID)
    |         % grid availability is gone
    |         y=1;
    |     end
    |     
    |     if (In.EEPROM.M1==1 && In.DCParams.Voc>SVocThresh+VocOffset)
    |         % auto mode and solar power is back
    |         y=1;
    |     end
    | end
  function dur=heaterDuration(TA):
    | function dur=heaterDuration(TA)
    |  
    | if TA<HeatTempThresh3
    |     % run for 30 min
    |     dur=30*60;
    | elseif TA<HeatTempThresh2
    |     dur=60*interp1([HeatTempThresh3 HeatTempThresh2],[30 5], TA);
    | else
    |     dur=60*interp1([HeatTempThresh2 HeatTempThresh1],[5 2], TA);
    | end
  function y=TempCondition(R, In):
    | function y=TempCondition(R, In)
    |  
    | % 0.5 is for Hysteresis in Temp Control
    | 
    | if (~R.FV)
    |     if (In.Sensors.TH1>T(In.EEPROM.B)+0.5)
    |         y=1;
    |     else
    |         y=0;
    |     end
    | else
    |     if (In.Sensors.TH1<(T(In.EEPROM.B)-0.5))
    |         y=0;
    |     else
    |         y=1;
    |     end
    | end
  function y = TV1TempOnCondition(R, In):
    | function y = TV1TempOnCondition(R, In)
    | 
    | % 0.5 ensures Hysteresis in Temp Control
    | 
    | if ~R.TV1
    |     if (max(In.Sensors.TES1,In.Sensors.TES2)>TSTempSetPoint+0.5)
    |         y=1;
    |     else
    |         y=0;
    |     end
    | else
    |     if (max(In.Sensors.TES1, In.Sensors.TES2)<TSTempSetPoint-0.5)
    |         y=0;
    |     else
    |         y=1;
    |     end
    | end
  function y=CDF2Condition(R, In):
    | function y=CDF2Condition(R, In)
    |  
    | if ((R.CRUN && In.Sensors.TA>CDF2TempThreshold && ~In.DCParams.F2_LPS) || In.DCParams.F1_HPS)
    |     y=1;
    | else
    |     y=0;
    | end
  function y=HCondition(In):
    | function y=HCondition(In)
    |  
    | if (In.Sensors.RH1<H(In.EEPROM.B))
    |     y=1;
    | else
    |     y=0;
    | end
  function y=powerOnCondition(R, In):
    | function y=powerOnCondition(R, In)
    |  
    | [~,y] = PowerModeSelection(R, In);
  function y=HCondition(In):
    | function y=HCondition(In)
    |  
    | if (In.Sensors.RH1<H(In.EEPROM.B))
    |     y=1;
    | else
    |     y=0;
    | end
  function y=TempCheck(R, In):
    | function y=TempCheck(R, In)
    |  
    | % 0.5 is for Hysteresis in Temp Control
    | 
    | if (~R.F1)
    |     if (In.Sensors.TH1>T(In.EEPROM.B)+1)
    |         y=1;
    |     else
    |         y=0;
    |     end
    | else
    |     if (In.Sensors.TH1<T(In.EEPROM.B))
    |         y=0;
    |     else
    |         y=1;
    |     end
    | end
  function y=powerOnCondition(R, In):
    | function y=powerOnCondition(R, In)
    |  
    | [~,y] = PowerModeSelection(R, In);
  function dur=heaterDuration(TA):
    | function dur=heaterDuration(TA)
    |  
    | if TA<HeatTempThresh3
    |     % run for 30 min
    |     dur=30*60;
    | elseif TA<HeatTempThresh2
    |     dur=60*interp1([HeatTempThresh3 HeatTempThresh2],[30 5], TA);
    | else
    |     dur=60*interp1([HeatTempThresh2 HeatTempThresh1],[5 2], TA);
    | end
  function y=TempCondition(R, In):
    | function y=TempCondition(R, In)
    |  
    | % 0.5 is for Hysteresis in Temp Control
    | 
    | if (~R.FV)
    |     if (In.Sensors.TH1>T(In.EEPROM.B)+2)
    |         y=1;
    |     else
    |         y=0;
    |     end
    | else
    |     if (In.Sensors.TH1<(T(In.EEPROM.B)-0.5))
    |         y=0;
    |     else
    |         y=1;
    |     end
    | end
  function y=CDF2Condition(R, In):
    | function y=CDF2Condition(R, In)
    |  
    | if ((R.CRUN && In.Sensors.TA>CDF2TempThreshold && ~In.DCParams.F2_LPS) || In.DCParams.F1_HPS)
    |     y=1;
    | else
    |     y=0;
    | end
  function y=HCondition(In):
    | function y=HCondition(In)
    |  
    | if (In.Sensors.RH1<H(In.EEPROM.B))
    |     y=1;
    | else
    |     y=0;
    | end
  function y=Diesel(R,In):
    | function y=Diesel(R,In)
    | if (In.Sensors.TH1>T(In.EEPROM.B)+2 && R.F1==0)
    |     y=1;
    | else
    |     y=0;
    | end
